simulink model "PlanControlZW_cs"  (R2020a)
settings: Solver=VariableStepAuto  StartTime=0.0  StopTime=100  FixedStep=1/1000  RelTol=1e-3
PreLoadFcn:
  | mbxruntime.callbacks.PreLoadFcn(bdroot);
PostLoadFcn:
  | mbxruntime.callbacks.PostLoadFcn(bdroot);
InitFcn:
  | mbxruntime.callbacks.InitFcn(bdroot);
StartFcn:
  | mbxruntime.callbacks.StartFcn(bdroot);
StopFcn:
  | mbxruntime.callbacks.StopFcn(bdroot);
model workspace (MAT data in the model file):
  mbox_table : object (value not decoded)
  model_closed = 0
  sim_status = 0
values from neighbouring files (symbols this model uses):
  c_factor = 43.75    [emplanner_init.m]
  cf = -175016    [emplanner_init.m]
  cr = -130634    [emplanner_init.m]
  global_path_x = [-2.22044604925e-16 0.999382255067 1.99750536558 2.99435224935 3.98991712279 4.98419835808 5.97719585569 6.96891007764 7.95934169183 8.94849144113 9.93636009523 10.9229484329 ... (501 elements, 501x1)]    [global_Path.mat]
  global_path_y = [-1.75 -1.75 -1.75 -1.75 -1.75 -1.75 -1.75 -1.75 -1.75 -1.75 -1.75 -1.75 ... (501 elements, 501x1)]    [global_Path.mat]
  KD_PID_distance = 0.0    (= 0)    [emplanner_init.m]
  KD_PID_speed = 0    [emplanner_init.m]
  KI_PID_distance = 0.0    (= 0)    [emplanner_init.m]
  KI_PID_speed = 0    [emplanner_init.m]
  KP_PID_distance = 0.5    [emplanner_init.m]
  KP_PID_speed = 1.8    [emplanner_init.m]
  la = 1.265    [emplanner_init.m]
  lb = 2.947-1.265    (= 1.682)    [emplanner_init.m]
  LQR_K1 = k(:,1)'    [emplanner_init.m]
  LQR_K2 = k(:,2)'    [emplanner_init.m]
  LQR_K3 = k(:,3)'    [emplanner_init.m]
  LQR_K4 = k(:,4)'    [emplanner_init.m]
  m = 2020    [emplanner_init.m]
  rack_displacement = [-39.14 , -37.2 , -35.29 , -33.43 , -31.6 , -29.81 , -28.06 , -26.34 , -24.66 ,      -23.01 , -21.38 , -19.79 , -18.23 , -16.69 , -15.18 , -13.7 , -12.23 , -10.8 , -9.38 , -7.98 ,     -6.61 , -5.25 , -3.91 , -2.59 , -1.29 , 0 , 1.27 , 2.54 , 3.78 , 5.02 , 6.24 , 7.46 , 8.66 ,      9.86 , 11.05 , 12.24 , 13.41 , 14.59 , 15.76 , 16.92 , 18.09 , 19.25 , 20.42 , 21.59 , 22.76 ,      23.93 , 25.11 , 26 ...(+26 chars)    [emplanner_init.m]
  refrence_path_x = [2.22044604925e-16 0.999382255067 1.99750536558 2.99435224935 3.98991712279 4.98419835808 5.97719585569 6.96891007764 7.95934169183 8.94849144113 9.93636009523 10.9229484329 ... (501 elements, 501x1)]    [refrence_path_two.mat]
  refrence_path_y = [1.75 1.75 1.75 1.75 1.75 1.75 1.75 1.75 1.75 1.75 1.75 1.75 ... (501 elements, 501x1)]    [refrence_path_two.mat]
  right_wheel_ground = [-70 ,-67.2 , -64.4 , -61.6 , -58.8 , -56 , -53.2 , -50.4 , -47.6 , -44.8 , -42 ,      -39.2 , -36.4 , -33.6 , -30.8 , -28 , -25.2 , -22.4 , -19.6 , -16.8 , -14 , -11.2 , -8.4 , -5.6 ,      -2.8 , 0 , 2.8 , 5.6 , 8.4 , 11.2 , 14 , 16.8 , 19.6 , 22.4 , 25.2 , 28 , 30.8 , 33.6 , 36.4 ,      39.2 , 42 , 44.8 , 47.6 , 50.4 , 53.2 , 56 , 58.8 , 61.6 , 64.4 , 67.2 , 70 ]    [emplanner_init.m]
  vx_break_point = zeros(1,5000)    [emplanner_init.m]
undefined symbols (not defined in the file or in its folder): aubr, DiscIntNeverNeededParam, tablebr, vubr
libraries: PreScanSimulinkLibrary x34, simulink_extras x5, Solver_SF x1
(part 4 of 10)

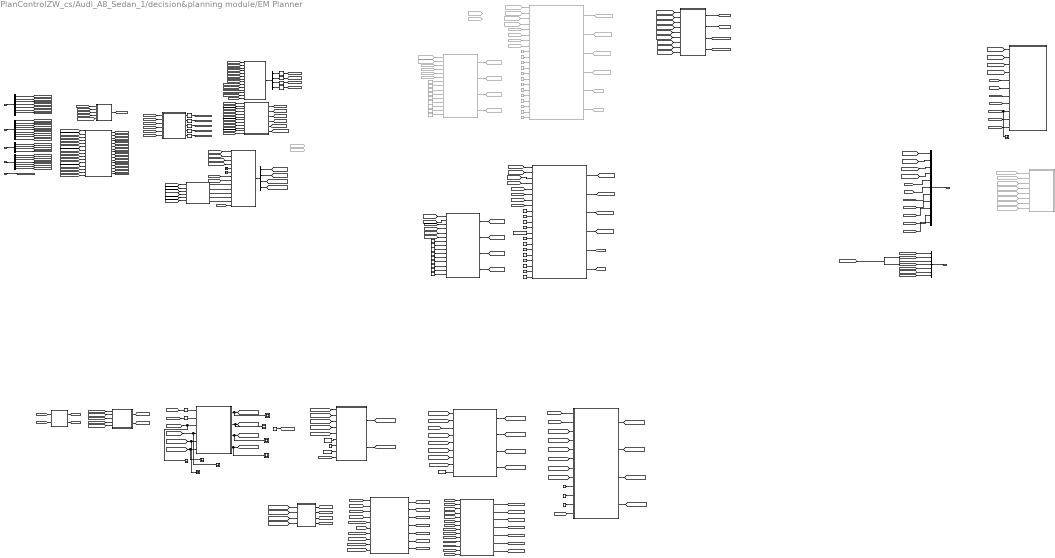
== system PlanControlZW_cs/Audi_A8_Sedan_1/decision&planning module/EM Planner ==
  referenceline info : Inport
  location info : Inport  Port=2
  perception info : Inport  Port=3
  pre_planning info : Inport  Port=4
  current time : Inport  Port=5
  Bus Creator : BusCreator  Inputs=7
  Bus Selector : BusSelector  OutputSignals=referenceline_x,referenceline_y,referenceline_heading,referenceline_kappa,origin_match_point_index,origin_x,origin_y
  Bus Selector1 : BusSelector  OutputSignals=host_x,host_y,host_heading_xy,host_vx,host_vy,host_yawrate,host_speed,host_ax,host_ay
  Bus Selector2 : BusSelector  OutputSignals=obs_x_set_gcs,obs_y_set_gcs,obs_velocity_set_gcs,obs_heading_set_gcs
  Bus Selector3 : BusSelector  OutputSignals=trajectory_x_gcs,trajectory_y_gcs,trajectory_heading_gcs,trajectory_kappa_gcs,trajectory_speed_gcs,trajectory_accel_gcs,trajectory_time_gcs
  Bus Selector4 : BusSelector  OutputSignals=s_set,l_set,dl_set,ddl_set
  Bus Selector5 : BusSelector  OutputSignals=s_set,l_set,s_dot_set,l_dot_set
  Cartesian2Frenet : Subsystem
  Cartesian2Frenet1 : Subsystem
  Constant : Constant  Commented=on  Value=1e6
  Constant1 : Constant  Commented=on  Value=2000
  Constant10 : Constant  Commented=on  Value=0.1
  Constant11 : Constant  Commented=on  Value=0.02
  Constant12 : Constant  Commented=on  Value=2
  Constant13 : Constant  Commented=on  Value=25000
  Constant14 : Constant  Commented=on  Value=50
  Constant15 : Constant  Commented=on  Value=20
  Constant{7,16..19} (5 alike) : Constant  Commented=on  Value=15
  Constant2 : Constant  Commented=on  Value=2
  Constant20 : Constant  Commented=on  Value=3
  Constant21 : Constant  Commented=on  Value=3
  Constant22 : Constant  Commented=on  Value=1.63
  Constant{23,39..41,50} (5 alike) : Constant  Value=15
  Constant24 : Constant  Value=400000
  Constant25 : Constant  Value=100
  Constant26 : Constant  Value=100
  Constant27 : Constant  Value=0.5*9.8
  Constant28 : Constant  Value=50
  Constant29 : Constant  Value=500
  Constant3 : Constant  Commented=on  Value=3
  Constant30 : Constant  Value=1e6
  Constant31 : Constant  Value=2000
  Constant32 : Constant  Value=0.5
  Constant33 : Constant  Value=0.2
  Constant34 : Constant  Value=2
  Constant35 : Constant  Value=25000
  Constant36 : Constant  Value=50
  Constant37 : Constant  Value=20
  Constant38 : Constant  Value=500
  Constant4 : Constant  Commented=on  Value=10
  Constant42 : Constant  Value=2
  Constant43 : Constant  Value=3
  Constant44 : Constant  Value=3
  Constant45 : Constant  Value=1.63
  Constant46 : Constant  Value=3
  Constant47 : Constant  Value=10
  Constant48 : Constant  Value=11
  Constant49 : Constant  Value=4
  Constant5 : Constant  Commented=on  Value=11
  Constant51 : Constant
  Constant6 : Constant  Commented=on  Value=4
  Constant8 : Constant  Commented=on
  Constant9 : Constant  Value=10
  Delay : Delay  DelayLength=1
  Delay1 : Delay  DelayLength=1
  Frenet2Cartesian task : MATLAB Function  TreatAsAtomicUnit=on
  From105 : From  Commented=on  GotoTag=dp_speed_s
  From106 : From  Commented=on  GotoTag=dp_speed_t
  From165 : From  Commented=on  GotoTag=obs_st_s_in_set
  From166 : From  Commented=on  GotoTag=obs_st_s_out_set
  From167 : From  Commented=on  GotoTag=obs_st_t_in_set
  From168 : From  Commented=on  GotoTag=obs_st_t_out_set
  From177 : From  Commented=on  GotoTag=qp_s_init
  From178 : From  Commented=on  GotoTag=relative_time_init
  From189 : From  Commented=on  GotoTag=dynamic_obs_s_set
  From190 : From  Commented=on  GotoTag=dynamic_obs_l_set
  From191 : From  Commented=on  GotoTag=dynamic_obs_s_set
  From192 : From  Commented=on  GotoTag=dynamic_obs_l_set
  From52 : From  Commented=on  GotoTag=static_obs_s_set
  From53 : From  Commented=on  GotoTag=static_obs_l_set
  From54 : From  Commented=on  GotoTag=plan_start_s
  From55 : From  Commented=on  GotoTag=plan_start_l
  From56 : From  Commented=on  GotoTag=plan_start_dl
  From57 : From  Commented=on  GotoTag=plan_start_ddl
  From58 : From  Commented=on  GotoTag=dp_path_s_final
  From59 : From  Commented=on  GotoTag=dp_path_l_final
  From60 : From  Commented=on  GotoTag=static_obs_s_set
  From61 : From  Commented=on  GotoTag=static_obs_l_set
  From62 : From  Commented=on  GotoTag=plan_start_l
  From63 : From  Commented=on  GotoTag=plan_start_dl
  From92 : From  Commented=on  GotoTag=plan_start_ddl
  From93 : From  Commented=on  GotoTag=plan_start_s
  Goto113 : Goto  Commented=on  GotoTag=l_min
  Goto114 : Goto  Commented=on  GotoTag=l_max
  Goto58 : Goto  Commented=on  GotoTag=dp_path_s_final
  Goto59 : Goto  Commented=on  GotoTag=dp_path_l_final
  Goto60 : Goto  Commented=on  GotoTag=dp_path_dl_final
  Goto61 : Goto  Commented=on  GotoTag=dp_path_ddl_final
  Goto89 : Goto  Commented=on  GotoTag=qp_path_s_final
  Goto90 : Goto  Commented=on  GotoTag=qp_path_l_final
  Goto91 : Goto  Commented=on  GotoTag=qp_path_dl_final
  Goto92 : Goto  Commented=on  GotoTag=qp_path_ddl_final
  Ground : Ground
  Ground1 : Ground
  MATLAB Function1 : MATLAB Function  TreatAsAtomicUnit=on
  MATLAB Function2 : MATLAB Function  TreatAsAtomicUnit=on
  MATLAB Function3 : MATLAB Function  TreatAsAtomicUnit=on
  MATLAB Function5 : MATLAB Function  Commented=on  TreatAsAtomicUnit=on
  Mux : Mux  Inputs=11
  Scope{,1..8} (9 alike) : Scope
  Selector{1..9} (9 alike) : Selector  InputPortWidth=128  IndexOptions=Index vector (dialog)  Indices=1  OutputSizes=1
  calc path length and map between point and s1 : MATLAB Function  TreatAsAtomicUnit=on
  calc plan start info and stitch trajectory : MATLAB Function  TreatAsAtomicUnit=on
  calc speed planning start condition1 : MATLAB Function  TreatAsAtomicUnit=on
  generate convex space : MATLAB Function  TreatAsAtomicUnit=on
  generate st graph : MATLAB Function  TreatAsAtomicUnit=on
  genrate index to s : MATLAB Function  TreatAsAtomicUnit=on
  increase st point count : MATLAB Function  TreatAsAtomicUnit=on
  obs : Subsystem
  path and speed merge : MATLAB Function  TreatAsAtomicUnit=on
  path decision task : Subsystem  Commented=on
  path decision task1 : Subsystem
  path planning task : Subsystem  Commented=on
  path planning task1 : Subsystem
  plot : MATLAB Function  TreatAsAtomicUnit=on
  spee planning with quadratic programming (qp) : MATLAB Function  TreatAsAtomicUnit=on
  speed decision with dynamic planning(dp) : MATLAB Function  TreatAsAtomicUnit=on
  stitch trajectory : MATLAB Function  TreatAsAtomicUnit=on
  EM Planner result : Outport
  result_plot_debug : Outport  Port=2
  wires:
  referenceline info/1 -> Bus Selector/1
  location info/1 -> Bus Selector1/1
  perception info/1 -> Bus Selector2/1
  pre_planning info/1 -> Bus Selector3/1
  current time/1 -> [current_time]
  Bus Selector3/1 -> [pre_trajectory_x_gcs]  "<trajectory_x_gcs>"
  Bus Selector3/2 -> [pre_trajectory_y_gcs]  "<trajectory_y_gcs>"
  Bus Selector3/3 -> [pre_trajectory_heading_gcs]  "<trajectory_heading_gcs>"
  Bus Selector3/4 -> [pre_trajectory_kappa_gcs]  "<trajectory_kappa_gcs>"
  Bus Selector3/5 -> [pre_trajectory_speed_gcs]  "<trajectory_speed_gcs>"
  Bus Selector3/6 -> [pre_trajectory_accel_gcs]  "<trajectory_accel_gcs>"
  Bus Selector3/7 -> [pre_trajectory_time]  "<trajectory_time_gcs>"
  Bus Selector2/1 -> [obs_x_set_gcs]  "<obs_x_set_gcs>"
  Bus Selector2/2 -> [obs_y_set_gcs]  "<obs_y_set_gcs>"
  Bus Selector2/3 -> [obs_velocity_set_gcs]  "<obs_velocity_set_gcs>"
  Bus Selector2/4 -> [obs_heading_set_gcs]  "<obs_heading_set_gcs>"
  Bus Selector1/1 -> [host_x]  "<host_x>"
  Bus Selector1/2 -> [host_y]  "<host_y>"
  Bus Selector1/3 -> [host_heading_xy]  "<host_heading_xy>"
  Bus Selector1/4 -> [host_vx_vcs]  "<host_vx>"
  Bus Selector1/5 -> [host_vy_vcs]  "<host_vy>"
  Bus Selector1/6 -> [host_yawrate]  "<host_yawrate>"
  Bus Selector1/7 -> [host_speed]  "<host_speed>"
  Bus Selector1/8 -> [host_ax_vcs]  "<host_ax>"
  Bus Selector1/9 -> [host_ay_vcs]  "<host_ay>"
  Bus Selector/1 -> [referenceline_x]  "<referenceline_x>"
  Bus Selector/2 -> [referenceline_y]  "<referenceline_y>"
  Bus Selector/3 -> [referenceline_heading]  "<referenceline_heading>"
  Bus Selector/4 -> [referenceline_kappa]  "<referenceline_kappa>"
  [host_ay_vcs] -> calc plan start info and stitch trajectory/15(host_ay)
  [host_ax_vcs] -> calc plan start info and stitch trajectory/14(host_ax)
  [host_vy_vcs] -> calc plan start info and stitch trajectory/13(host_vy)
  [host_vx_vcs] -> calc plan start info and stitch trajectory/12(host_vx)
  [host_heading_xy] -> calc plan start info and stitch trajectory/11(host_heading_xy)
  [host_y] -> calc plan start info and stitch trajectory/10(host_y)
  [host_x] -> calc plan start info and stitch trajectory/9(host_x)
  [current_time] -> calc plan start info and stitch trajectory/8(current_time)
  [pre_trajectory_x_gcs] -> calc plan start info and stitch trajectory/1(pre_trajectory_x)
  [pre_trajectory_y_gcs] -> calc plan start info and stitch trajectory/2(pre_trajectory_y)
  [pre_trajectory_time] -> calc plan start info and stitch trajectory/7(pre_trajectory_time)
  [pre_trajectory_accel_gcs] -> calc plan start info and stitch trajectory/6(pre_trajectory_accel)
  [pre_trajectory_speed_gcs] -> calc plan start info and stitch trajectory/5(pre_trajectory_velocity)
  [pre_trajectory_kappa_gcs] -> calc plan start info and stitch trajectory/4(pre_trajectory_kappa)
  [pre_trajectory_heading_gcs] -> calc plan start info and stitch trajectory/3(pre_trajectory_heading)
  calc plan start info and stitch trajectory/1(plan_start_x) -> [plan_start_x_gcs]
  calc plan start info and stitch trajectory/2(plan_start_y) -> [plan_start_y_gcs]
  calc plan start info and stitch trajectory/3(plan_start_heading) -> [plan_start_heading_gcs]
  calc plan start info and stitch trajectory/4(plan_start_kappa) -> [plan_start_kappa_gcs]
  calc plan start info and stitch trajectory/5(plan_start_vx) -> [plan_start_vx_gcs]
  calc plan start info and stitch trajectory/6(plan_start_vy) -> [plan_start_vy_gcs]
  calc plan start info and stitch trajectory/7(plan_start_ax) -> [plan_start_ax_gcs]
  calc plan start info and stitch trajectory/8(plan_start_ay) -> [plan_start_ay_gcs]
  calc plan start info and stitch trajectory/9(plan_start_time) -> [plan_start_time]
  calc plan start info and stitch trajectory/10(stitch_x) -> [stitch_x_gcs]
  calc plan start info and stitch trajectory/11(stitch_y) -> [stitch_y_gcs]
  calc plan start info and stitch trajectory/12(stitch_heading) -> [stitch_heading_gcs]
  calc plan start info and stitch trajectory/13(stitch_kappa) -> [stitch_kappa_gcs]
  calc plan start info and stitch trajectory/14(stitch_speed) -> [stitch_speed_gcs]
  calc plan start info and stitch trajectory/15(stitch_accel) -> [stitch_accel_gcs]
  calc plan start info and stitch trajectory/16(stitch_time) -> [stitch_time]
  Bus Selector/5 -> [origin_match_point_index]  "<origin_match_point_index>"
  Bus Selector/6 -> [origin_x]  "<origin_x>"
  Bus Selector/7 -> [origin_y]  "<origin_y>"
  [referenceline_x] -> genrate index to s/1(path_x)
  [referenceline_y] -> genrate index to s/2(path_y)
  [origin_x] -> genrate index to s/3(origin_x)
  [origin_y] -> genrate index to s/4(origin_y)
  [origin_match_point_index] -> genrate index to s/5(origin_match_point_index)
  genrate index to s/1(index2s) -> [index2s]
  MATLAB Function2/5(proj_kappa_set) -> Selector5/1
  MATLAB Function2/3(proj_y_set) -> Selector3/1
  MATLAB Function2/1(match_point_index_set) -> Selector1/1
  MATLAB Function2/4(proj_heading_set) -> Selector4/1
  MATLAB Function2/2(proj_x_set) -> Selector2/1
  [plan_start_x_gcs] -> MATLAB Function2/1(x_set)
  [plan_start_y_gcs] -> MATLAB Function2/2(y_set)
  [referenceline_x] -> MATLAB Function2/3(frenet_path_x)
  [referenceline_y] -> MATLAB Function2/4(frenet_path_y)
  [referenceline_heading] -> MATLAB Function2/5(frenet_path_heading)
  [referenceline_kappa] -> MATLAB Function2/6(frenet_path_kappa)
  Selector1/1 -> [plan_start_match_point_index]
  Selector2/1 -> [plan_start_proj_x]
  Selector3/1 -> [plan_start_proj_y]
  Selector4/1 -> [plan_start_proj_heading]
  Selector5/1 -> [plan_start_proj_kappa]
  [plan_start_y_gcs] -> Cartesian2Frenet/2(y_set)
  [plan_start_x_gcs] -> Cartesian2Frenet/1(x_set)
  [plan_start_vx_gcs] -> Cartesian2Frenet/3(vx_set)
  [plan_start_vy_gcs] -> Cartesian2Frenet/4(vy_set)
  [plan_start_ax_gcs] -> Cartesian2Frenet/5(ax_set)
  [plan_start_ay_gcs] -> Cartesian2Frenet/6(ay_set)
  [referenceline_x] -> Cartesian2Frenet/7(frenet_path_x)
  [referenceline_y] -> Cartesian2Frenet/8(frenet_path_y)
  [plan_start_match_point_index] -> Cartesian2Frenet/9(proj_match_point_index_set)
  [plan_start_proj_x] -> Cartesian2Frenet/10(proj_x_set)
  [plan_start_proj_y] -> Cartesian2Frenet/11(proj_y_set)
  [plan_start_proj_heading] -> Cartesian2Frenet/12(proj_heading_set)
  [plan_start_proj_kappa] -> Cartesian2Frenet/13(proj_kappa_set)
  Cartesian2Frenet/1(Cartesian2FrenetOut) -> Bus Selector4/1
  Bus Selector4/4 -> Selector9/1  "<ddl_set>"
  Bus Selector4/3 -> Selector8/1  "<dl_set>"
  Bus Selector4/2 -> Selector7/1  "<l_set>"
  Bus Selector4/1 -> Selector6/1  "<s_set>"
  Selector6/1 -> [plan_start_s]
  Selector7/1 -> [plan_start_l]
  Selector8/1 -> [plan_start_dl]
  Selector9/1 -> [plan_start_ddl]
  [index2s] -> Cartesian2Frenet/14(index2s)
  [host_x] -> obs/1(host_x)
  [host_y] -> obs/2(host_y)
  [host_heading_xy] -> obs/3(host_heading_xy)
  [obs_x_set_gcs] -> obs/4(obs_x_set_gcs)
  [obs_y_set_gcs] -> obs/5(obs_y_set_gcs)
  [obs_velocity_set_gcs] -> obs/6(obs_velocity_set_gcs)
  [obs_heading_set_gcs] -> obs/7(obs_heading_set_gcs)
  [referenceline_x] -> obs/8(referenceline_x)
  [referenceline_y] -> obs/9(referenceline_y)
  [referenceline_heading] -> obs/10(referenceline_heading)
  [referenceline_kappa] -> obs/11(referenceline_kappa)
  [index2s] -> obs/12(index2s)
  obs/1(static_obs_s_set) -> [static_obs_s_set]
  obs/5(dynamic_obs_vx_set) -> [dynamic_obs_vx_set]
  Bus Creator/1 -> EM Planner result/1
  [trajectory_x_final] -> Bus Creator/1  "trajectory_x_gcs"
  [trajectory_time_final] -> Bus Creator/7  "trajectory_time_gcs"
  [trajectory_accel_final] -> Bus Creator/6  "trajectory_accel_gcs"
  [trajectory_speed_final] -> Bus Creator/5  "trajectory_speed_gcs"
  [trajectory_heading_final] -> MATLAB Function1/1(trajectory_heading_final)  "trajectory_heading_gcs"
  [trajectory_kappa_final] -> Bus Creator/4  "trajectory_kappa_gcs"
  [trajectory_y_final] -> Bus Creator/2  "trajectory_y_gcs"
  From55/1 -> path decision task/4(plan_start_l)
  Constant5/1 -> path decision task/12(dp_row)
  path decision task/4(dp_path_ddl_final) -> Goto61/1
  Constant3/1 -> path decision task/10(dp_cost_dddl)
  Constant1/1 -> path decision task/8(dp_cost_dl)
  Constant4/1 -> path decision task/11(dp_cost_ref)
  path decision task/1(dp_path_s_final) -> Goto58/1
  Constant2/1 -> path decision task/9(dp_cost_ddl)
  Constant8/1 -> path decision task/15(dp_sample_l)
  From54/1 -> path decision task/3(plan_start_s)
  Constant7/1 -> path decision task/14(dp_sample_s)
  From57/1 -> path decision task/6(plan_start_ddl)
  From56/1 -> path decision task/5(plan_start_dl)
  Constant/1 -> path decision task/7(dp_cost_collision)
  From190/1 -> path decision task/2(static_obs_l_set)
  From189/1 -> path decision task/1(static_obs_s_set)
  path decision task/3(dp_path_dl_final) -> Goto60/1
  path decision task/2(dp_path_l_final) -> Goto59/1
  Constant6/1 -> path decision task/13(dp_col)
  From191/1 -> path planning task/3(static_obs_s_set)
  Constant22/1 -> path planning task/19(host_w)
  path planning task/4(qp_path_ddl_final) -> Goto92/1
  From63/1 -> path planning task/7(plan_start_dl)
  From92/1 -> path planning task/8(plan_start_ddl)
  From192/1 -> path planning task/4(static_obs_l_set)
  From59/1 -> path planning task/2(dp_path_l_final)
  Constant13/1 -> path planning task/10(qp_cost_dl)
  Constant12/1 -> path planning task/9(qp_cost_l)
  path planning task/3(qp_path_dl_final) -> Goto91/1
  path planning task/1(qp_path_s_final) -> Goto89/1
  From58/1 -> path planning task/1(dp_path_s_final)
  Constant10/1 -> path planning task/20(delta_dl_max)
  Constant11/1 -> path planning task/21(delta_ddl_max)
  Constant17/1 -> path planning task/14(qp_cost_endl)
  From93/1 -> path planning task/5(plan_start_s)
  Constant20/1 -> path planning task/17(host_d1)
  Constant18/1 -> path planning task/15(qp_cost_end_dl)
  Constant16/1 -> path planning task/13(qp_cost_centre)
  Constant15/1 -> path planning task/12(qp_cost_dddl)
  path planning task/2(qp_path_l_final) -> Goto90/1
  Constant19/1 -> path planning task/16(qp_cost_end_ddl)
  From62/1 -> path planning task/6(plan_start_l)
  Constant21/1 -> path planning task/18(host_d2)
  Constant14/1 -> path planning task/11(qp_cost_ddl)
  [dp_path_l_final] -> plot/2(dp_l)
  [plan_start_s] -> plot/9(start_s), Scope8/1
  [l_min] -> plot/5(l_min)
  [qp_path_l_final] -> plot/4(qp_l)
  [l_max] -> plot/6(l_max)
  [static_obs_s_set] -> plot/7(obs_s_set)
  [dp_path_s_final] -> plot/1(dp_s)
  [static_obs_l_set] -> plot/8(obs_l_set)
  [plan_start_l] -> plot/10(start_l)
  [plan_start_dl] -> plot/11(start_dl)
  [qp_path_s_final] -> plot/3(qp_s)
  Frenet2Cartesian task/1(x_set) -> [trajectory_x_init]
  [qp_path_s_final] -> Frenet2Cartesian task/1(s_set)
  [referenceline_kappa] -> Frenet2Cartesian task/8(frenet_path_kappa)
  [qp_path_dl_final] -> Frenet2Cartesian task/3(dl_set)
  [qp_path_ddl_final] -> Frenet2Cartesian task/4(ddl_set)
  [index2s] -> Frenet2Cartesian task/9(index2s)
  [qp_path_l_final] -> Frenet2Cartesian task/2(l_set)
  Frenet2Cartesian task/3(heading_set) -> [trajectory_heading_init]
  Frenet2Cartesian task/2(y_set) -> [trajectory_y_init]
  [referenceline_y] -> Frenet2Cartesian task/6(frenet_path_y)
  [referenceline_x] -> Frenet2Cartesian task/5(frenet_path_x)
  Frenet2Cartesian task/4(kappa_set) -> [trajectory_kappa_init]
  [referenceline_heading] -> Frenet2Cartesian task/7(frenet_path_heading)
  MATLAB Function1/1(y) -> Bus Creator/3  "trajectory_heading_gcs"
  obs/2(static_obs_l_set) -> [static_obs_l_set]
  obs/3(dynamic_obs_x_set) -> [dynamic_obs_x_set]
  obs/4(dynamic_obs_y_set) -> [dynamic_obs_y_set]
  obs/6(dynamic_obs_vy_set) -> [dynamic_obs_vy_set]
  calc path length and map between point and s1/1(path_s_end) -> [path_s_end]
  [trajectory_y_init] -> calc path length and map between point and s1/2(trajectory_y)
  calc path length and map between point and s1/2(path_index2s) -> [path_index2s]
  [trajectory_x_init] -> calc path length and map between point and s1/1(trajectory_x)
  Ground1/1 -> Cartesian2Frenet1/6(ay_set)
  MATLAB Function3/4(proj_heading_set) -> Cartesian2Frenet1/12(proj_heading_set)
  MATLAB Function3/3(proj_y_set) -> Cartesian2Frenet1/11(proj_y_set)
  Bus Selector5/2 -> [dynamic_obs_l_set]  "<l_set>"
  Cartesian2Frenet1/1(Cartesian2FrenetOut) -> Bus Selector5/1
  Bus Selector5/4 -> [dynamic_obs_l_dot_set]  "<l_dot_set>"
  Bus Selector5/1 -> [dynamic_obs_s_set]  "<s_set>"
  MATLAB Function3/1(match_point_index_set) -> Cartesian2Frenet1/9(proj_match_point_index_set)
  MATLAB Function3/5(proj_kappa_set) -> Cartesian2Frenet1/13(proj_kappa_set)
  MATLAB Function3/2(proj_x_set) -> Cartesian2Frenet1/10(proj_x_set)
  Ground/1 -> Cartesian2Frenet1/5(ax_set)
  Bus Selector5/3 -> [dynamic_obs_s_dot_set]  "<s_dot_set>"
  [dynamic_obs_y_set] -> Cartesian2Frenet1/2(y_set)
  [trajectory_y_init] -> Cartesian2Frenet1/8(frenet_path_y)
  [path_index2s] -> Cartesian2Frenet1/14(index2s)
  [dynamic_obs_x_set] -> Cartesian2Frenet1/1(x_set)
  [trajectory_x_init] -> Cartesian2Frenet1/7(frenet_path_x)
  [dynamic_obs_vx_set] -> Cartesian2Frenet1/3(vx_set)
  [dynamic_obs_vy_set] -> Cartesian2Frenet1/4(vy_set)
  [dynamic_obs_x_set] -> MATLAB Function3/1(x_set)
  [trajectory_y_init] -> MATLAB Function3/4(frenet_path_y)
  [trajectory_kappa_init] -> MATLAB Function3/6(frenet_path_kappa)
  [dynamic_obs_y_set] -> MATLAB Function3/2(y_set)
  [trajectory_x_init] -> MATLAB Function3/3(frenet_path_x)
  [trajectory_heading_init] -> MATLAB Function3/5(frenet_path_heading)
  [plan_start_vy_gcs] -> calc speed planning start condition1/2(plan_start_vy)
  [plan_start_ax_gcs] -> calc speed planning start condition1/3(plan_start_ax)
  calc speed planning start condition1/1(plan_start_s_dot) -> [plan_start_s_dot]
  calc speed planning start condition1/2(plan_start_s_dot2) -> [plan_start_s_dot2]
  [plan_start_vx_gcs] -> calc speed planning start condition1/1(plan_start_vx)
  [plan_start_ay_gcs] -> calc speed planning start condition1/4(plan_start_ay)
  [plan_start_heading_gcs] -> calc speed planning start condition1/5(plan_start_heading)
  [s] -> Delay/1
  Delay1/1 -> generate st graph/2(pre_trajectory_t)
  [dynamic_obs_s_dot_set] -> Scope6/1, generate st graph/5(dynamic_obs_s_dot_set)
  generate st graph/2(obs_st_s_out_set) -> Scope3/1, [obs_st_s_out_set]
  generate st graph/3(obs_st_t_in_set) -> Scope2/1, [obs_st_t_in_set]
  [dynamic_obs_l_set] -> Scope5/1, generate st graph/4(dynamic_obs_l_set)
  Delay/1 -> generate st graph/1(pre_trajectory_s)
  generate st graph/1(obs_st_s_in_set) -> Scope4/1, [obs_st_s_in_set]
  [dynamic_obs_l_dot_set] -> Scope/1, generate st graph/6(dynamic_obs_l_dot_set)
  [dynamic_obs_s_set] -> Scope7/1, generate st graph/3(dynamic_obs_s_set)
  [relative_time] -> Delay1/1
  generate st graph/4(obs_st_t_out_set) -> Scope1/1, [obs_st_t_out_set]
  Constant23/1 -> [reference_speed]
  Constant26/1 -> speed decision with dynamic planning(dp)/8(w_cost_obs)
  [plan_start_s_dot] -> speed decision with dynamic planning(dp)/9(plan_start_s_dot)
  [obs_st_s_in_set] -> speed decision with dynamic planning(dp)/1(obs_st_s_in_set)
  Constant24/1 -> speed decision with dynamic planning(dp)/6(w_cost_ref_speed)
  speed decision with dynamic planning(dp)/2(dp_speed_t) -> [dp_speed_t]
  Constant25/1 -> speed decision with dynamic planning(dp)/7(w_cost_accel)
  [obs_st_t_out_set] -> speed decision with dynamic planning(dp)/4(obs_st_t_out_set)
  speed decision with dynamic planning(dp)/1(dp_speed_s) -> [dp_speed_s]
  [obs_st_s_out_set] -> speed decision with dynamic planning(dp)/2(obs_st_s_out_set)
  [obs_st_t_in_set] -> speed decision with dynamic planning(dp)/3(obs_st_t_in_set)
  [reference_speed] -> speed decision with dynamic planning(dp)/5(reference_speed_unlimit)
  [trajectory_kappa_init] -> generate convex space/8(trajectory_kappa_init)
  [obs_st_s_out_set] -> generate convex space/5(obs_st_s_out_set)
  [dp_speed_t] -> generate convex space/2(dp_speed_t)
  [path_index2s] -> generate convex space/3(path_index2s)
  [s_ub] -> spee planning with quadratic programming (qp)/6(s_ub)
  [dp_speed_s] -> spee planning with quadratic programming (qp)/3(dp_speed_s)
  generate convex space/2(s_ub) -> [s_ub]
  generate convex space/4(s_dot_ub) -> [s_dot_ub]
  Constant27/1 -> generate convex space/9(max_lateral_accel)
  generate convex space/3(s_dot_lb) -> [s_dot_lb]
  [s_lb] -> spee planning with quadratic programming (qp)/5(s_lb)
  [s_dot_lb] -> spee planning with quadratic programming (qp)/7(s_dot_lb)
  [obs_st_t_out_set] -> generate convex space/7(obs_st_t_out_set)
  [obs_st_s_in_set] -> generate convex space/4(obs_st_s_in_set)
  Constant28/1 -> spee planning with quadratic programming (qp)/10(w_cost_v_ref)
  [reference_speed] -> spee planning with quadratic programming (qp)/12(speed_reference)
  generate convex space/1(s_lb) -> [s_lb]
  spee planning with quadratic programming (qp)/3(qp_s_dot2_init) -> [qp_s_dot2_init]
  [plan_start_s_dot] -> spee planning with quadratic programming (qp)/1(plan_start_s_dot)
  Constant29/1 -> spee planning with quadratic programming (qp)/11(w_cost_jerk)
  [dp_speed_s] -> generate convex space/1(dp_speed_s)
  spee planning with quadratic programming (qp)/2(qp_s_dot_init) -> [qp_s_dot_init]
  spee planning with quadratic programming (qp)/1(qp_s_init) -> [qp_s_init]
  [s_dot_ub] -> spee planning with quadratic programming (qp)/8(s_dot_ub)
  [obs_st_t_in_set] -> generate convex space/6(obs_st_t_in_set)
  [plan_start_s_dot2] -> spee planning with quadratic programming (qp)/2(plan_start_s_dot2)
  [dp_speed_t] -> spee planning with quadratic programming (qp)/4(dp_speed_t)
  Constant9/1 -> spee planning with quadratic programming (qp)/9(w_cost_s_dot2)
  spee planning with quadratic programming (qp)/4(relative_time_init) -> [relative_time_init]
  [stitch_heading_gcs] -> stitch trajectory/10(stitch_heading)
  [stitch_speed_gcs] -> stitch trajectory/12(stitch_speed)
  stitch trajectory/7(trajectory_time_final) -> [trajectory_time_final]
  [trajectory_x_init] -> path and speed merge/7(trajectory_x_init)
  [stitch_x_gcs] -> stitch trajectory/8(stitch_x)
  [qp_s_dot2_init] -> increase st point count/3(s_dot2_init)
  stitch trajectory/2(trajectory_y_final) -> [trajectory_y_final]
  stitch trajectory/6(trajectory_accel_final) -> [trajectory_accel_final]
  path and speed merge/6(trajectory_accel) -> [trajectory_accel]
  [trajectory_accel] -> stitch trajectory/6(trajectory_accel)
  [trajectory_heading_init] -> path and speed merge/9(trajectory_heading_init)
  [qp_s_init] -> increase st point count/1(s_init)
  [relative_time_init] -> increase st point count/4(relative_time_init)
  [trajectory_heading] -> stitch trajectory/3(trajectory_heading)
  [s_dot] -> path and speed merge/2(s_dot)
  stitch trajectory/1(trajectory_x_final) -> [trajectory_x_final]
  increase st point count/4(relative_time) -> [relative_time]
  increase st point count/1(s) -> [s]
  increase st point count/2(s_dot) -> [s_dot]
  [trajectory_time] -> stitch trajectory/7(trajectory_time)
  [path_index2s] -> path and speed merge/6(path_s)
  stitch trajectory/4(trajectory_kappa_final) -> [trajectory_kappa_final]
  [stitch_time] -> stitch trajectory/14(stitch_time)
  [trajectory_x] -> stitch trajectory/1(trajectory_x)
  path and speed merge/4(trajectory_kappa) -> [trajectory_kappa]
  path and speed merge/5(trajectory_speed) -> [trajectory_speed]
  [plan_start_time] -> path and speed merge/5(current_time)
  path and speed merge/2(trajectory_y) -> [trajectory_y]
  [qp_s_dot_init] -> increase st point count/2(s_dot_init)
  [stitch_kappa_gcs] -> stitch trajectory/11(stitch_kappa)
  increase st point count/3(s_dot2) -> [s_dot2]
  [stitch_accel_gcs] -> stitch trajectory/13(stitch_accel)
  [relative_time] -> path and speed merge/4(relative_time)
  [trajectory_kappa_init] -> path and speed merge/10(trajectory_kappa_init)
  stitch trajectory/3(trajectory_heading_final) -> [trajectory_heading_final]
  [s_dot2] -> path and speed merge/3(s_dot2)
  [trajectory_y] -> stitch trajectory/2(trajectory_y)
  [trajectory_speed] -> stitch trajectory/5(trajectory_speed)
  [stitch_y_gcs] -> stitch trajectory/9(stitch_y)
  path and speed merge/7(trajectory_time) -> [trajectory_time]
  path and speed merge/1(trajectory_x) -> [trajectory_x]
  [trajectory_kappa] -> stitch trajectory/4(trajectory_kappa)
  stitch trajectory/5(trajectory_speed_final) -> [trajectory_speed_final]
  path and speed merge/3(trajectory_heading) -> [trajectory_heading]
  [s] -> path and speed merge/1(s)
  [trajectory_y_init] -> path and speed merge/8(trajectory_y_init)
  From166/1 -> MATLAB Function5/6(obs_s_out_set)
  From106/1 -> MATLAB Function5/2(dp_speed_t)
  From168/1 -> MATLAB Function5/8(obs_t_out_set)
  From167/1 -> MATLAB Function5/7(obs_t_in_set)
  From177/1 -> MATLAB Function5/3(qp_speed_s)
  From165/1 -> MATLAB Function5/5(obs_s_in_set)
  From105/1 -> MATLAB Function5/1(dp_speed_s)
  From178/1 -> MATLAB Function5/4(qp_speed_t)
  path planning task/5(l_min) -> Goto113/1
  path planning task/6(l_max) -> Goto114/1
  [dp_path_s_final] -> Mux/1
  [dp_path_l_final] -> Mux/2
  [qp_path_s_final] -> Mux/3
  [qp_path_l_final] -> Mux/4
  [l_min] -> Mux/5
  [l_max] -> Mux/6
  [static_obs_s_set] -> Mux/7
  [static_obs_l_set] -> Mux/8
  [plan_start_s] -> Mux/9
  [plan_start_l] -> Mux/10
  [plan_start_dl] -> Mux/11
  Mux/1 -> result_plot_debug/1
  [static_obs_l_set] -> path decision task1/2(static_obs_l_set)
  [plan_start_ddl] -> path decision task1/6(plan_start_ddl)
  Constant46/1 -> path decision task1/10(dp_cost_dddl)
  Constant51/1 -> path decision task1/15(dp_sample_l)
  Constant50/1 -> path decision task1/14(dp_sample_s)
  path planning task1/6(l_max) -> [l_max]
  Constant38/1 -> path planning task1/13(qp_cost_centre)
  [dp_path_s_final] -> path planning task1/1(dp_path_s_final)
  Constant45/1 -> path planning task1/19(host_w)
  Constant37/1 -> path planning task1/12(qp_cost_dddl)
  path planning task1/4(qp_path_ddl_final) -> [qp_path_ddl_final]
  Constant41/1 -> path planning task1/16(qp_cost_end_ddl)
  path planning task1/2(qp_path_l_final) -> [qp_path_l_final]
  Constant40/1 -> path planning task1/15(qp_cost_end_dl)
  path decision task1/2(dp_path_l_final) -> [dp_path_l_final]
  Constant49/1 -> path decision task1/13(dp_col)
  [plan_start_l] -> path planning task1/6(plan_start_l)
  Constant44/1 -> path planning task1/18(host_d2)
  Constant43/1 -> path planning task1/17(host_d1)
  Constant42/1 -> path decision task1/9(dp_cost_ddl)
  Constant30/1 -> path decision task1/7(dp_cost_collision)
  path decision task1/3(dp_path_dl_final) -> [dp_path_dl_final]
  [plan_start_dl] -> path planning task1/7(plan_start_dl)
  [plan_start_s] -> path planning task1/5(plan_start_s)
  Constant35/1 -> path planning task1/10(qp_cost_dl)
  [dp_path_l_final] -> path planning task1/2(dp_path_l_final)
  Constant31/1 -> path decision task1/8(dp_cost_dl)
  path planning task1/5(l_min) -> [l_min]
  Constant39/1 -> path planning task1/14(qp_cost_endl)
  path planning task1/3(qp_path_dl_final) -> [qp_path_dl_final]
  [plan_start_ddl] -> path planning task1/8(plan_start_ddl)
  Constant34/1 -> path planning task1/9(qp_cost_l)
  Constant48/1 -> path decision task1/12(dp_row)
  Constant32/1 -> path planning task1/20(delta_dl_max)
  [static_obs_s_set] -> path decision task1/1(static_obs_s_set)
  [plan_start_s] -> path decision task1/3(plan_start_s)
  Constant36/1 -> path planning task1/11(qp_cost_ddl)
  [plan_start_dl] -> path decision task1/5(plan_start_dl)
  Constant33/1 -> path planning task1/21(delta_ddl_max)
  [plan_start_l] -> path decision task1/4(plan_start_l)
  Constant47/1 -> path decision task1/11(dp_cost_ref)
  path planning task1/1(qp_path_s_final) -> [qp_path_s_final]
  path decision task1/1(dp_path_s_final) -> [dp_path_s_final]
  path decision task1/4(dp_path_ddl_final) -> [dp_path_ddl_final]
  [static_obs_l_set] -> path planning task1/4(static_obs_l_set)
  [static_obs_s_set] -> path planning task1/3(static_obs_s_set)

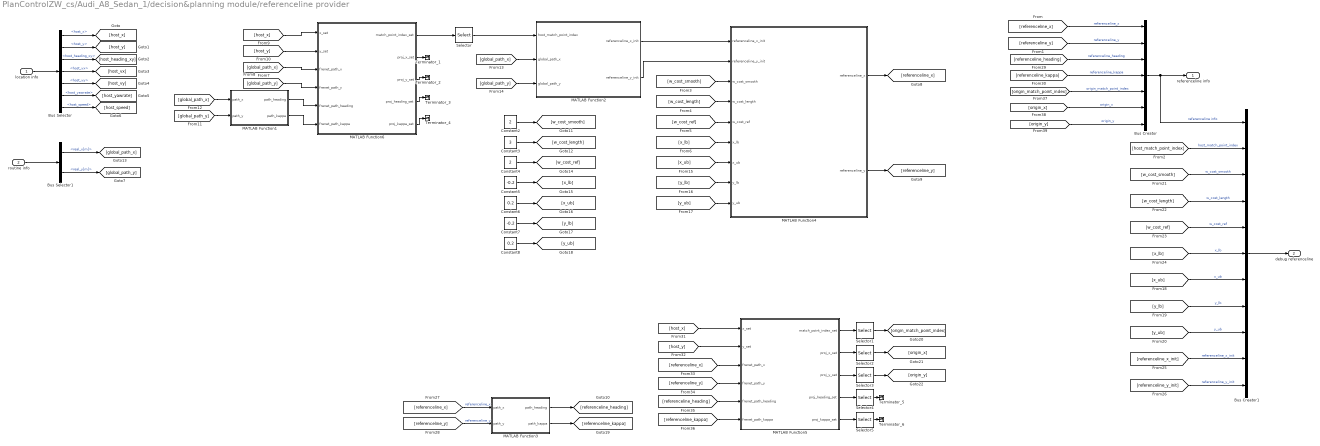
== system PlanControlZW_cs/Audi_A8_Sedan_1/decision&planning module/referenceline provider ==
  location info : Inport
  routine info : Inport  Port=2
  Bus Creator : BusCreator  Inputs=7
  Bus Creator1 : BusCreator  Inputs=11
  Bus Selector : BusSelector  OutputSignals=host_x,host_y,host_heading_xy,host_vx,host_vy,host_yawrate,host_speed
  Bus Selector1 : BusSelector  OutputSignals=real_x[m],real_y[m]
  Constant2 : Constant  Value=2
  Constant3 : Constant  Value=3
  Constant4 : Constant  Value=2
  Constant5 : Constant  Value=-0.2
  Constant6 : Constant  Value=0.2
  Constant7 : Constant  Value=-0.2
  Constant8 : Constant  Value=0.2
  MATLAB Function1 : MATLAB Function  TreatAsAtomicUnit=on
  MATLAB Function2 : MATLAB Function  TreatAsAtomicUnit=on
  MATLAB Function3 : MATLAB Function  TreatAsAtomicUnit=on
  MATLAB Function4 : MATLAB Function  TreatAsAtomicUnit=on
  MATLAB Function5 : MATLAB Function  TreatAsAtomicUnit=on
  MATLAB Function6 : MATLAB Function  TreatAsAtomicUnit=on
  Selector{,1..5} (6 alike) : Selector  InputPortWidth=128  IndexOptions=Index vector (dialog)  Indices=1  OutputSizes=1
  Terminator_{1..6} (6 alike) : Terminator
  referenceline info : Outport
  debug referenceline : Outport  Port=2
  wires:
  [global_path_x] -> MATLAB Function2/2(global_path_x)
  [host_x] -> MATLAB Function6/1(x_set)
  MATLAB Function1/2(path_kappa) -> MATLAB Function6/6(frenet_path_kappa)
  MATLAB Function1/1(path_heading) -> MATLAB Function6/5(frenet_path_heading)
  [global_path_y] -> MATLAB Function6/4(frenet_path_y)
  [global_path_x] -> MATLAB Function6/3(frenet_path_x)
  [host_y] -> MATLAB Function6/2(y_set)
  [global_path_y] -> MATLAB Function1/2(path_y)
  [global_path_x] -> MATLAB Function1/1(path_x)
  Selector/1 -> MATLAB Function2/1(host_match_point_index)
  MATLAB Function6/1(match_point_index_set) -> Selector/1
  [global_path_y] -> MATLAB Function2/3(global_path_y)
  MATLAB Function2/1(referenceline_x_init) -> MATLAB Function4/1(referenceline_x_init)
  Bus Selector/5 -> [host_vy]  "<host_vy>"
  Bus Selector/1 -> [host_x]  "<host_x>"
  Bus Selector/2 -> [host_y]  "<host_y>"
  Bus Selector/3 -> [host_heading_xy]  "<host_heading_xy>"
  Bus Selector/4 -> [host_vx]  "<host_vx>"
  Bus Selector/7 -> [host_speed]  "<host_speed>"
  Bus Selector/6 -> [host_yawrate]  "<host_yawrate>"
  location info/1 -> Bus Selector/1
  Bus Selector1/2 -> [global_path_y]  "<real_y[m]>"
  Bus Selector1/1 -> [global_path_x]  "<real_x[m]>"
  routine info/1 -> Bus Selector1/1
  MATLAB Function4/1(referenceline_x) -> [referenceline_x]
  MATLAB Function4/2(referenceline_y) -> [referenceline_y]
  [referenceline_x] -> Bus Creator/1  "referenceline_x"
  [referenceline_y] -> Bus Creator/2  "referenceline_y"
  Bus Creator1/1 -> debug referenceline/1
  Bus Creator/1 -> Bus Creator1/1, referenceline info/1  "referenceline info"
  Constant2/1 -> [w_cost_smooth]
  Constant3/1 -> [w_cost_length]
  Constant8/1 -> [y_ub]
  Constant7/1 -> [y_lb]
  Constant6/1 -> [x_ub]
  Constant5/1 -> [x_lb]
  Constant4/1 -> [w_cost_ref]
  [w_cost_smooth] -> MATLAB Function4/3(w_cost_smooth)
  [w_cost_length] -> MATLAB Function4/4(w_cost_length)
  [w_cost_ref] -> MATLAB Function4/5(w_cost_ref)
  [x_lb] -> MATLAB Function4/6(x_lb)
  [x_ub] -> MATLAB Function4/7(x_ub)
  [y_lb] -> MATLAB Function4/8(y_lb)
  [y_ub] -> MATLAB Function4/9(y_ub)
  MATLAB Function2/2(referenceline_y_init) -> MATLAB Function4/2(referenceline_y_init)
  [w_cost_ref] -> Bus Creator1/5  "w_cost_ref"
  [x_lb] -> Bus Creator1/6  "x_lb"
  [w_cost_length] -> Bus Creator1/4  "w_cost_length"
  [x_ub] -> Bus Creator1/7  "x_ub"
  [w_cost_smooth] -> Bus Creator1/3  "w_cost_smooth"
  [y_lb] -> Bus Creator1/8  "y_lb"
  [host_match_point_index] -> Bus Creator1/2  "host_match_point_index"
  [y_ub] -> Bus Creator1/9  "y_ub"
  [referenceline_x_init] -> Bus Creator1/10  "referenceline_x_init"
  [referenceline_y_init] -> Bus Creator1/11  "referenceline_y_init"
  MATLAB Function6/2(proj_x_set) -> Terminator_1/1
  MATLAB Function6/3(proj_y_set) -> Terminator_2/1
  MATLAB Function6/4(proj_heading_set) -> Terminator_3/1
  MATLAB Function6/5(proj_kappa_set) -> Terminator_4/1
  Selector5/1 -> Terminator_6/1
  Selector1/1 -> [origin_match_point_index]
  Selector4/1 -> Terminator_5/1
  MATLAB Function5/5(proj_kappa_set) -> Selector5/1
  Selector2/1 -> [origin_x]
  MATLAB Function5/1(match_point_index_set) -> Selector1/1
  MATLAB Function5/3(proj_y_set) -> Selector3/1
  MATLAB Function5/4(proj_heading_set) -> Selector4/1
  MATLAB Function5/2(proj_x_set) -> Selector2/1
  [host_x] -> MATLAB Function5/1(x_set)
  Selector3/1 -> [origin_y]
  MATLAB Function3/1(path_heading) -> [referenceline_heading]
  MATLAB Function3/2(path_kappa) -> [referenceline_kappa]
  [referenceline_y] -> MATLAB Function3/2(path_y)  "referenceline_y"
  [referenceline_x] -> MATLAB Function3/1(path_x)  "referenceline_x"
  [referenceline_heading] -> Bus Creator/3  "referenceline_heading"
  [referenceline_kappa] -> Bus Creator/4  "referenceline_kappa"
  [origin_match_point_index] -> Bus Creator/5  "origin_match_point_index"
  [origin_x] -> Bus Creator/6  "origin_x"
  [origin_y] -> Bus Creator/7  "origin_y"
  [host_y] -> MATLAB Function5/2(y_set)
  [referenceline_x] -> MATLAB Function5/3(frenet_path_x)
  [referenceline_y] -> MATLAB Function5/4(frenet_path_y)
  [referenceline_heading] -> MATLAB Function5/5(frenet_path_heading)
  [referenceline_kappa] -> MATLAB Function5/6(frenet_path_kappa)

== system PlanControlZW_cs/BMW_X5_SUV_1/SELF_Demux/compas converter ==
  rotz [rad] : Inport
  cart2compas : Subsystem
  rad2deg : Gain  Gain=180/pi
  heading [deg] : Outport
  wires:
  rad2deg/1 -> cart2compas/1(Angle [deg])
  rotz [rad]/1 -> rad2deg/1
  cart2compas/1(heading [deg]) -> heading [deg]/1

== system PlanControlZW_cs/BMW_X5_SUV_1/Trajectories/Traj2State1 ==
  Traj Org : Inport
  Offset : Inport  Port=2
  Add2 : Sum
  ApplyRotation : PreScanSimulinkLibrary/ApplyRotation  SystemSampleTime=-1  Latency=0  AutoFrameSizeCalculation=off
  ApplyRotation1 : PreScanSimulinkLibrary/ApplyRotation  SystemSampleTime=-1  Latency=0  AutoFrameSizeCalculation=off
  ApplyRotation2 : PreScanSimulinkLibrary/ApplyRotation  SystemSampleTime=-1  Latency=0  AutoFrameSizeCalculation=off
  Constant : Constant  Value=zeros(12,1)
  Mux : Mux  Inputs=6
  Mux1 : Mux  Inputs=2
  Mux{2,4..9} (7 alike) : Mux  Inputs=3
  Mux3 : Mux  Inputs=2
  Selector : Selector  InputPortWidth=6  IndexOptions=Index vector (dialog)  Indices=[4 5 6]  OutputSizes=1
  Selector1 : Selector  InputPortWidth=21  IndexOptions=Index vector (dialog)  Indices=[5]  OutputSizes=1
  Selector10 : Selector  InputPortWidth=21  IndexOptions=Index vector (dialog)  Indices=[2]  OutputSizes=1
  Selector11 : Selector  InputPortWidth=21  IndexOptions=Index vector (dialog)  Indices=[3]  OutputSizes=1
  Selector12 : Selector  InputPortWidth=21  IndexOptions=Index vector (dialog)  Indices=[1]  OutputSizes=1
  Selector13 : Selector  InputPortWidth=21  IndexOptions=Index vector (dialog)  Indices=[8]  OutputSizes=1
  Selector14 : Selector  InputPortWidth=21  IndexOptions=Index vector (dialog)  Indices=[9]  OutputSizes=1
  Selector15 : Selector  InputPortWidth=21  IndexOptions=Index vector (dialog)  Indices=[7]  OutputSizes=1
  Selector16 : Selector  InputPortWidth=21  IndexOptions=Index vector (dialog)  Indices=[14]  OutputSizes=1
  Selector17 : Selector  InputPortWidth=21  IndexOptions=Index vector (dialog)  Indices=[15]  OutputSizes=1
  Selector18 : Selector  InputPortWidth=21  IndexOptions=Index vector (dialog)  Indices=[13]  OutputSizes=1
  Selector19 : Selector  InputPortWidth=21  IndexOptions=Index vector (dialog)  Indices=[20]  OutputSizes=1
  Selector2 : Selector  InputPortWidth=21  IndexOptions=Index vector (dialog)  Indices=[6]  OutputSizes=1
  Selector20 : Selector  InputPortWidth=21  IndexOptions=Index vector (dialog)  Indices=[21]  OutputSizes=1
  Selector21 : Selector  InputPortWidth=21  IndexOptions=Index vector (dialog)  Indices=[19]  OutputSizes=1
  Selector3 : Selector  InputPortWidth=21  IndexOptions=Index vector (dialog)  Indices=[12]  OutputSizes=1
  Selector4 : Selector  InputPortWidth=21  IndexOptions=Index vector (dialog)  Indices=[17]  OutputSizes=1
  Selector5 : Selector  InputPortWidth=21  IndexOptions=Index vector (dialog)  Indices=[18]  OutputSizes=1
  Selector6 : Selector  InputPortWidth=21  IndexOptions=Index vector (dialog)  Indices=[16]  OutputSizes=1
  Selector7 : Selector  InputPortWidth=21  IndexOptions=Index vector (dialog)  Indices=[11]  OutputSizes=1
  Selector8 : Selector  InputPortWidth=21  IndexOptions=Index vector (dialog)  Indices=[10]  OutputSizes=1
  Selector9 : Selector  InputPortWidth=21  IndexOptions=Index vector (dialog)  Indices=[4]  OutputSizes=1
  Traj2State2 : Subsystem
  state : Outport
  wires:
  Mux9/1 -> ApplyRotation2/2, ApplyRotation1/2, ApplyRotation/2
  Selector20/1 -> Mux9/3
  Selector19/1 -> Mux9/2
  Selector21/1 -> Mux9/1
  Selector5/1 -> Mux8/3
  Selector4/1 -> Mux8/2
  Selector6/1 -> Mux8/1
  Mux8/1 -> Mux/6
  Mux6/1 -> ApplyRotation2/1
  Mux7/1 -> Mux/4
  ApplyRotation2/1 -> Mux/5
  Selector3/1 -> Mux7/3
  Selector7/1 -> Mux7/2
  Selector8/1 -> Mux7/1
  Mux4/1 -> Mux/2
  Mux5/1 -> ApplyRotation1/1
  ApplyRotation1/1 -> Mux/3
  Mux2/1 -> ApplyRotation/1
  ApplyRotation/1 -> Mux/1
  Selector2/1 -> Mux4/3
  Selector1/1 -> Mux4/2
  Selector9/1 -> Mux4/1
  Selector17/1 -> Mux6/3
  Selector16/1 -> Mux6/2
  Selector18/1 -> Mux6/1
  Selector14/1 -> Mux5/3
  Selector13/1 -> Mux5/2
  Selector15/1 -> Mux5/1
  Selector11/1 -> Mux2/3
  Selector10/1 -> Mux2/2
  Selector12/1 -> Mux2/1
  Mux3/1 -> Selector8/1, Selector7/1, Selector3/1, Selector18/1, Selector16/1, Selector17/1, Selector6/1, Selector20/1, Selector19/1, Selector21/1, Selector5/1, Selector4/1, Selector14/1, Selector13/1, Selector15/1, Selector2/1, Selector1/1, Selector9/1, Selector12/1, Selector10/1, Selector11/1
  Mux1/1 -> Add2/2
  Constant/1 -> Mux1/2
  Add2/1 -> Traj2State2/1(traj)
  Selector/1 -> Mux3/2
  Traj Org/1 -> Mux3/1
  Offset/1 -> Mux1/1, Selector/1
  Mux/1 -> Add2/1
  Traj2State2/1(state) -> state/1

== system PlanControlZW_cs/BMW_X5_SUV_1/Trajectories/TrajCoGOffset ==
  State In : Inport
  Add : Sum  Inputs=+-+
  Add1 : Sum
  ApplyRotation : PreScanSimulinkLibrary/ApplyRotation  SystemSampleTime=-1  Latency=0  AutoFrameSizeCalculation=off
  ApplyRotation1 : PreScanSimulinkLibrary/ApplyRotation  SystemSampleTime=-1  Latency=0  AutoFrameSizeCalculation=off
  CoG Offset : Constant  Value=[0 0 CoGOffsetZ]
  Degrees to Radians : simulink_extras/Transformations/Degrees to Radians
  Demux1 : Demux  Outputs=[3 3 3]
  Mux : Mux  Inputs=[3 3 3]
  Orientation : Constant  Value=[InitRoll InitPitch 0]
  State Out : Outport
  wires:
  State In/1 -> Demux1/1
  Demux1/1 -> Add/1
  Add/1 -> Mux/1
  Demux1/3 -> Mux/3, Add1/2
  Mux/1 -> State Out/1
  Demux1/2 -> Mux/2
  Orientation/1 -> Degrees to Radians/1
  ApplyRotation/1 -> Add/3
  ApplyRotation1/1 -> Add/2
  Add1/1 -> ApplyRotation/2
  CoG Offset/1 -> ApplyRotation1/1, ApplyRotation/1
  Degrees to Radians/1 -> Add1/1, ApplyRotation1/2

== system PlanControlZW_cs/BMW_X5_SUV_1/Trajectories/Trajectory_3 ==
  From Workspace : FromWorkspace  VariableName=trajectory  SampleTime=TimeStep  ZeroCross=off  OutputAfterFinalValue=Holding final value
  From Workspace1 : FromWorkspace  VariableName=trajectory  SampleTime=TimeStep  ZeroCross=off  OutputAfterFinalValue=Setting to zero
  Mux : Mux  Inputs=2
  Selector1 : Selector  InputPortWidth=24  IndexOptions=Index vector (dialog)  Indices=[7:18]  OutputSizes=1
  Selector9 : Selector  InputPortWidth=24  IndexOptions=Index vector (dialog)  Indices=[1:6]  OutputSizes=1
  trajectory : Outport
  wires:
  From Workspace/1 -> Selector9/1
  From Workspace1/1 -> Selector1/1
  Mux/1 -> trajectory/1
  Selector9/1 -> Mux/1
  Selector1/1 -> Mux/2

== system PlanControlZW_cs/Box_1/Dynamics_Empty/MuxState ==
  note: mode: Dynamics
  note: mode: Positioning
  note: mode: Dynamics
      | VelVEHICLE
      | wrt VEH
  note: AnglesVEHICLE
      | wrtGLOB
  note: For state mode 'Dynamic' positions
      | are not taken into account, as they
      | are computed by integrating velocity.
      | Click annotation for Help.
  x [m] : Inport  SampleTime=TimeStep
  y [m] : Inport  Port=2  SampleTime=TimeStep
  z [m] : Inport  Port=3  SampleTime=TimeStep
  dx [m/s] : Inport  Port=4  SampleTime=TimeStep
  dy [m/s] : Inport  Port=5  SampleTime=TimeStep
  dz [m/s] : Inport  Port=6  SampleTime=TimeStep
  R [rad] : Inport  Port=7  SampleTime=TimeStep
  P [rad] : Inport  Port=8  SampleTime=TimeStep
  Y [rad] : Inport  Port=9  SampleTime=TimeStep
  Constant : Constant  DisableCoverage=on  Value=positioningmode
  Discrete-Time Integrator : DiscreteIntegrator  SampleTime=TimeStep  ICPrevOutput=DiscIntNeverNeededParam  ICPrevScaledInput=DiscIntNeverNeededParam
  Ground : Ground
  Ground1 : Ground
  Mux1 : Mux  Inputs=[3 3]
  Mux2 : Mux  Inputs=3
  Mux3 : Mux  Inputs=3
  Mux4 : Mux  Inputs=3
  Mux5 : Mux  Inputs=[3 3]
  Mux6 : Mux  Inputs=[6 3]
  Switch : Switch  Threshold=0.5
  Transformation_BODY2GLOBAL : PreScanSimulinkLibrary/Simple_Vehicle_Dynamics/Chassis/MuxDynState/Transformation_BODY2GLOBAL  SystemSampleTime=-1  Latency=0  AutoFrameSizeCalculation=off
  mux3 : Mux  Inputs=3
  state : Outport
  wires:
  Constant/1 -> Switch/2
  Mux6/1 -> state/1
  Mux4/1 -> Mux1/1
  Mux5/1 -> Switch/3
  Mux1/1 -> Switch/1
  Switch/1 -> Mux6/1  "PosVeh wrt  GLOB"
  P [rad]/1 -> Mux3/2
  R [rad]/1 -> Mux3/1
  dz [m/s]/1 -> Mux2/3
  dy [m/s]/1 -> Mux2/2
  dx [m/s]/1 -> Mux2/1
  z [m]/1 -> Mux4/3
  y [m]/1 -> Mux4/2
  x [m]/1 -> Mux4/1
  Ground1/1 -> mux3/2  "pitch"
  Y [rad]/1 -> mux3/3, Mux3/3  "yaw"
  Mux3/1 -> Mux6/2
  Transformation_BODY2GLOBAL/1 -> Discrete-Time Integrator/1, Mux5/2  "VelVEH wrt  GLOB"
  mux3/1 -> Transformation_BODY2GLOBAL/2
  Ground/1 -> mux3/1  "roll"
  Mux2/1 -> Mux1/2, Transformation_BODY2GLOBAL/1
  Discrete-Time Integrator/1 -> Mux5/1  "PosVEH wrt  GLOB"

== system PlanControlZW_cs/Box_1/SELF_Demux/compas converter ==
  rotz [rad] : Inport
  cart2compas : Subsystem
  rad2deg : Gain  Gain=180/pi
  heading [deg] : Outport
  wires:
  rad2deg/1 -> cart2compas/1(Angle [deg])
  rotz [rad]/1 -> rad2deg/1
  cart2compas/1(heading [deg]) -> heading [deg]/1

== system PlanControlZW_cs/Citroen_C3_Hatchback_1/SELF_Demux/compas converter ==
  rotz [rad] : Inport
  cart2compas : Subsystem
  rad2deg : Gain  Gain=180/pi
  heading [deg] : Outport
  wires:
  rad2deg/1 -> cart2compas/1(Angle [deg])
  rotz [rad]/1 -> rad2deg/1
  cart2compas/1(heading [deg]) -> heading [deg]/1
